simulink model "ecu1vib"  (Simulink 8.1)
settings: Solver=ode45  StartTime=0.0  StopTime=400  FixedStep=.01  RelTol=1e-3
undefined symbols (not defined in the file or in its folder): P, S
settings Model: Creator=Daniel  LastModifiedBy=Daniel
settings DataIOCC: SignalLoggingSaveFormat=Dataset
settings DebuggingCC: SolverPrmCheckMsg=none  FcnCallInpInsideContextMsg=EnableAllAsError
settings GRTTargetCC: CombineOutputUpdateFcns=on  GRTInterface=off

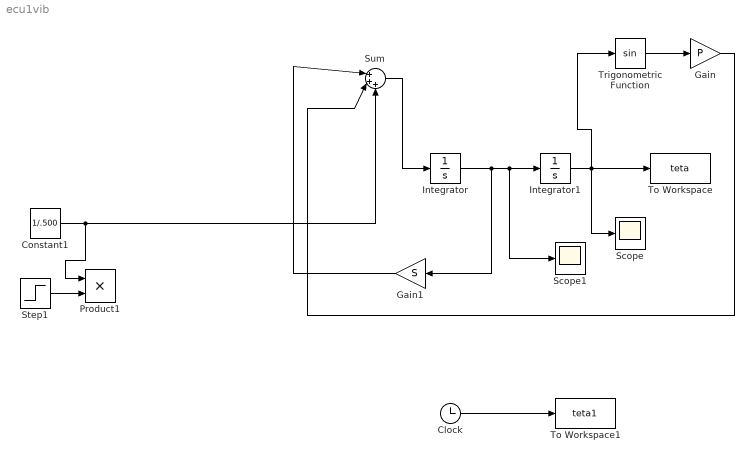
== system ecu1vib ==
  Clock : Clock
  Constant1 : Constant  Value=1/.500
  Gain : Gain  Gain=P
  Gain1 : Gain  Gain=S
  Integrator : Integrator
  Integrator1 : Integrator
  Product1 : Product
  Scope : Scope
      settings: SaveName=mio
  Scope1 : Scope
  Step1 : Step  SampleTime=0
  Sum : Sum  Inputs=|+++
  To Workspace : ToWorkspace  VariableName=teta  SampleTime=-1
  To Workspace1 : ToWorkspace  VariableName=teta1  SampleTime=-1
  Trigonometric Function : Trigonometry
  wires:
  Integrator1/1 -> Scope/1, To Workspace/1, Trigonometric Function/1
  Trigonometric Function/1 -> Gain/1
  Integrator/1 -> Gain1/1, Scope1/1, Integrator1/1
  Gain/1 -> Sum/2
  Clock/1 -> To Workspace1/1
  Gain1/1 -> Sum/1
  Sum/1 -> Integrator/1
  Constant1/1 -> Sum/3, Product1/1
  Step1/1 -> Product1/2
